simulink model "cpu2"  (R2020a)
settings: Solver=VariableStepAuto  StartTime=0.0  StopTime=10.0  RelTol=1e-3
libraries: simulink_extras x402, msbPllFoundation x1
(part 1 of 63)
settings Model: Creator=kishan  LastModifiedBy=kishan

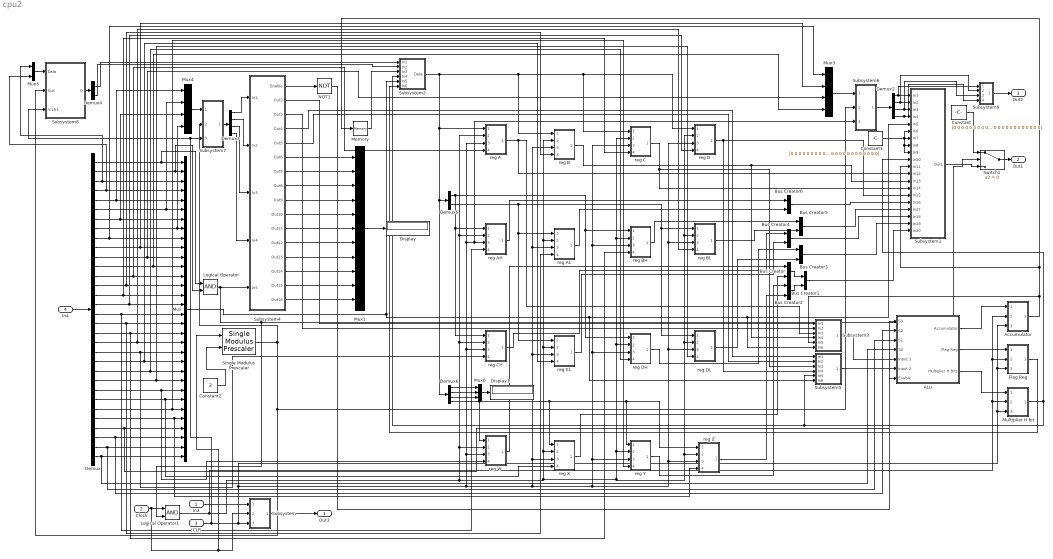
== system cpu2 ==
  In3 : Inport  OutDataTypeStr=boolean
  Clock : Inport  Port=2  OutDataTypeStr=boolean
  !CLR : Inport  Port=3  OutDataTypeStr=boolean
  In4 : Inport  Port=4
  ALU : Subsystem
  Accumulator : Subsystem
  Bus Creator{,1..6} (7 alike) : BusCreator  Inputs=2
  Constant : Constant  Value=[0 0 0 0 0 0 0 0 0 0 0 0 0 0 0 0 0 0 0 0 0 0 0 0 0 0 0 0 0 0 0 0]  OutDataTypeStr=boolean
  Constant1 : Constant  Value=[0 0 0 0 0 0 0 0 0 0 0 0 0 0 0 0 0 0 0 0 0 0 0 0 0 0 0 0 0 0 0 0]  OutDataTypeStr=boolean
  Constant2 : Constant  Value=2  OutDataTypeStr=double
  Demux : Demux  Outputs=32
  Demux2 : Demux
  Demux3 : Demux
  Demux4 : Demux  Outputs=2
  Demux5 : Demux  Outputs=2
  Demux6 : Demux
  Display : Display
  Display1 : Display
  Flag Reg : Subsystem
  Logical Operator : Logic  AllPortsSameDT=off  OutDataTypeStr=boolean
  Logical Operator1 : Logic  AllPortsSameDT=off  OutDataTypeStr=boolean
  Memory : Memory  InitialCondition=[0 0 0 0 0 0 0 0 0 0 0 0 0 0 0 0 0 0 0 0 0 0 0 0 0 0 0 0 0 0 0 0]
  Multiplier H bit : Subsystem
  Mux : Mux  Inputs=32
  Mux1 : Mux  Inputs=11
  Mux3 : Mux
  Mux4 : Mux
  Mux5 : Mux  Inputs=2
  Mux6 : Mux  Inputs=3
  NOT1 : Logic  Operator=NOT  IconShape=distinctive  AllPortsSameDT=off  OutDataTypeStr=boolean
  Single Modulus Prescaler : msbPllFoundation/Single Modulus Prescaler  ExtraBuffer=off  NBuffer=1
      settings: SourceProductBaseCode=AM
  Subsystem : Subsystem
  Subsystem1 : Subsystem
  Subsystem2 : Subsystem
  Subsystem3 : Subsystem
  Subsystem4 : Subsystem
  Subsystem5 : Subsystem
  Subsystem6 : Subsystem
  Subsystem7 : Subsystem
  Subsystem8 : Subsystem
  Subsystem9 : Subsystem
  Switch1 : Switch  Criteria=u2 > Threshold  OutDataTypeStr=boolean
  reg A : Subsystem
  reg AH : Subsystem
  reg AL : Subsystem
  reg B : Subsystem
  reg BH : Subsystem
  reg BL : Subsystem
  reg C : Subsystem
  reg CH : Subsystem
  reg CL : Subsystem
  reg D : Subsystem
  reg DH : Subsystem
  reg DL : Subsystem
  reg W : Subsystem
  reg X : Subsystem
  reg Y : Subsystem
  reg Z : Subsystem
  Out3 : Outport
  Out1 : Outport  Port=2
  Out2 : Outport  Port=3
  wires:
  Logical Operator/1 -> Logical Operator1/2, Switch1/2, Subsystem4/5(In5)
  Subsystem4/5(Out5) -> Subsystem5/2(In2)
  Demux/7 -> Mux/7, Mux4/3
  Demux/19 -> reg BH/4(Mux_in), Mux/19
  Mux/1 -> Subsystem5/6(In6), Subsystem3/6(In6), Subsystem1/5(In5), Subsystem2/5(In5)
  Subsystem5/1(Input 2) -> ALU/6(Input 2)
  Subsystem4/8(Out8) -> Mux1/3
  Subsystem4/13(Out13) -> Mux1/8
  Demux/23 -> reg DH/4(Mux_in), Mux/23
  Subsystem4/2(Out2) -> Subsystem3/1(In1)
  Accumulator/1(Out1) -> Memory/1, Subsystem1/11(In11), Subsystem3/5(In5)
  ALU/3(Multiplier H Bits) -> Multiplier H bit/1(In1)
  reg Y/1(Out1) -> Bus Creator2/1
  Demux/31 -> ALU/3(S1), Mux/31
  ALU/1(Accumulator) -> Accumulator/1(In1)
  reg Z/1(Out1) -> Bus Creator2/2
  Subsystem4/3(Out3) -> Subsystem3/2(In2)
  NOT1/1 -> ALU/7(Enable)
  Constant/1 -> Switch1/1
  Flag Reg/1(Out1) -> Subsystem2/6(In6)
  Bus Creator1/1 -> Subsystem1/20(In20)
  Demux/3 -> Mux5/1, Mux/3
  Demux/28 -> reg Z/4(Mux_in), Mux/28
  Clock/1 -> Single Modulus Prescaler/1, Subsystem/2(Clock), Logical Operator1/1
  Subsystem/1(Out1) -> Out3/1
  Subsystem4/15(Out15) -> Mux1/10
  Bus Creator/1 -> Bus Creator1/1
  reg B/1(Out1) -> Subsystem1/13(In13), Subsystem3/4(In4)
  reg AH/1(Out1) -> Bus Creator6/1
  Subsystem2/1(Data) -> reg D/1(Data), reg C/1(Data), reg B/1(Data), Demux6/1, Demux5/1, reg A/1(Data)
  Subsystem4/9(Out9) -> Mux1/4
  Demux/24 -> reg DL/4(Mux_in), Mux/24
  Demux/27 -> reg Y/4(Mux_in), Mux/27
  Subsystem4/1(Enable) -> NOT1/1
  reg C/1(Out1) -> Subsystem1/14(In14), Subsystem5/3(In3)
  Bus Creator6/1 -> Subsystem1/16(In16)
  reg BL/1(Out1) -> Bus Creator5/2
  In4/1 -> Demux/1
  Subsystem4/10(Out10) -> Mux1/5
  Subsystem4/7(Out7) -> Mux1/2
  reg DL/1(Out1) -> Bus Creator3/2
  Logical Operator1/1 -> Accumulator/2(In2), Flag Reg/2(In2), Multiplier H bit/2(In2), reg DH/2(In2), reg BH/2(In2), reg C/2(In2), reg Y/2(In2), reg Z/2(In2), reg BL/2(In2), reg D/2(In2), reg DL/2(In2), reg X/2(In2), reg CL/2(In2), reg AL/2(In2), reg B/2(In2), reg W/2(In2), reg CH/2(In2), reg AH/2(In2), reg A/2(In2)
  Bus Creator3/1 -> Subsystem1/19(In19)
  ALU/2(Flag Reg) -> Flag Reg/1(In1)
  reg W/1(Out1) -> Bus Creator/1
  Demux/15 -> reg C/4(Mux_in), Mux/15
  Demux/13 -> reg A/4(Mux_in), Mux/13
  In3/1 -> Subsystem/1(Interrupt)
  Demux/16 -> reg D/4(Mux_in), Mux/16
  Subsystem4/11(Out11) -> Mux1/6
  Bus Creator5/1 -> Subsystem1/17(In17)
  Subsystem4/14(Out14) -> Mux1/9
  Subsystem4/16(Out16) -> Mux1/11
  Demux/29 -> ALU/1(S3), Mux/29
  Subsystem4/12(Out12) -> Mux1/7
  reg D/1(Out1) -> Subsystem1/15(In15), Subsystem5/4(In4)
  Switch1/1 -> Out1/1
  Demux/11 -> Mux3/3, Mux/11
  Demux/2 -> Logical Operator/2, Mux/2
  reg CL/1(Out1) -> Bus Creator4/2
  Demux/5 -> Mux4/1, Mux/5
  Demux/20 -> reg BL/4(Mux_in), Mux/20
  Bus Creator4/1 -> Subsystem1/18(In18)
  Demux/9 -> Mux3/1, Mux/9
  Demux/1 -> Mux/1, Logical Operator/1
  Demux/14 -> reg B/4(Mux_in), Mux/14
  Demux/25 -> reg W/4(Mux_in), Mux/25
  Memory/1 -> Subsystem2/3(In3)
  Demux/26 -> reg X/4(Mux_in), Mux/26
  Demux/32 -> ALU/4(S0), Mux/32
  reg DH/1(Out1) -> Bus Creator3/1
  Demux/30 -> ALU/2(S2), Mux/30
  Multiplier H bit/1(Out1) -> Subsystem5/5(In5), Subsystem2/4(In4), Subsystem1/10(In10)
  Demux/6 -> Mux4/2, Mux/6
  Subsystem3/1(Input 1) -> ALU/5(Input 1)
  Subsystem4/6(Out6) -> Mux1/1
  Demux/10 -> Mux3/2, Mux/10
  Demux/12 -> Mux3/4, Mux/12
  Mux1/1 -> Display/1
  reg X/1(Out1) -> Bus Creator/2
  !CLR/1 -> Subsystem8/3(!CLR1), Subsystem7/3(!CLR), Accumulator/3(In3), Flag Reg/3(In3), Multiplier H bit/3(In3), reg CH/3(In3), Subsystem6/3(!CLR), reg AH/3(In3), reg A/3(In3), reg W/3(In3), reg X/3(In3), reg CL/3(In3), reg AL/3(In3), reg B/3(In3), reg DH/3(In3), reg BH/3(In3), reg C/3(In3), reg Y/3(In3), reg Z/3(In3), reg BL/3(In3), reg D/3(In3), reg DL/3(In3), Subsystem/3(Reset)
  reg A/1(Out1) -> Subsystem3/3(In3), Subsystem1/12(In12)
  Demux/8 -> Mux4/4, Mux/8
  Bus Creator2/1 -> Bus Creator1/2
  Subsystem4/4(Out4) -> Subsystem5/1(In1)
  Constant1/1 -> Subsystem1/9(In9), Subsystem1/8(In8), Subsystem1/7(In7), Subsystem1/6(In6)
  reg CH/1(Out1) -> Bus Creator4/1
  reg AL/1(Out1) -> Bus Creator6/2
  reg BH/1(Out1) -> Bus Creator5/1
  Demux/22 -> reg CL/4(Mux_in), Mux/22
  Demux/21 -> reg CH/4(Mux_in), Mux/21
  Demux/4 -> Mux5/2, Mux/4
  Demux/18 -> reg AL/4(Mux_in), Mux/18
  Subsystem1/1(Out1) -> Switch1/3
  Demux/17 -> reg AH/4(Mux_in), Mux/17
  Single Modulus Prescaler/1 -> Subsystem7/2(CLK), Subsystem8/2(CLK), Subsystem6/2(CLK)
  Constant2/1 -> Single Modulus Prescaler/2
  Mux3/1 -> Subsystem6/1(Data)
  Demux2/1 -> Subsystem1/1(In1), Subsystem9/1(In1)
  Demux2/2 -> Subsystem9/2(In2), Subsystem1/2(In2)
  Demux2/3 -> Subsystem9/3(In3), Subsystem1/3(In3)
  Demux2/4 -> Subsystem9/4(In4), Subsystem1/4(In4)
  Subsystem6/1(Out1) -> Demux2/1
  Subsystem7/1(Out1) -> Demux3/1
  Mux4/1 -> Subsystem7/1(Data)
  Demux3/1 -> Subsystem4/1(In1)
  Demux3/2 -> Subsystem4/2(In2)
  Demux3/4 -> Subsystem4/4(In4)
  Demux3/3 -> Subsystem4/3(In3)
  Mux5/1 -> Subsystem8/1(Data)
  Subsystem8/1(Q) -> Demux4/1
  Demux4/1 -> Subsystem2/1(In1)
  Demux4/2 -> Subsystem2/2(In2)
  Demux5/1 -> reg DH/1(Data), reg BH/1(Data), reg CH/1(Data), reg AH/1(Data)
  Demux5/2 -> reg DL/1(Data), reg BL/1(Data), reg CL/1(Data), reg AL/1(Data)
  Demux6/4 -> reg W/1(Data), reg X/1(Data), reg Y/1(Data), reg Z/1(Data)
  Demux6/1 -> Mux6/1
  Demux6/2 -> Mux6/2
  Demux6/3 -> Mux6/3
  Mux6/1 -> Display1/1
  Subsystem9/1(Out1) -> Out2/1

== system cpu2/ALU ==
  S3 : Inport
  S2 : Inport  Port=2
  S1 : Inport  Port=3
  S0 : Inport  Port=4
  Input 1 : Inport  Port=5
  Input 2 : Inport  Port=6
  Enable : Inport  Port=7
  Adder : Subsystem
  Comparartor : Subsystem
  Decrementer : Subsystem
  Demux : Demux  Outputs=32
  Demux1 : Demux  Outputs=32
  Incrementer : Subsystem
  Left Rotator : Subsystem
  Left shifter : Subsystem
  Logical Operator : Logic  AllPortsSameDT=off  OutDataTypeStr=boolean
  Logical Operator1 : Logic  Operator=OR  AllPortsSameDT=off  OutDataTypeStr=boolean
  Logical Operator2 : Logic  Operator=NOT  AllPortsSameDT=off  OutDataTypeStr=boolean
  Logical Operator4 : Logic  Operator=NOR  Inputs=32  AllPortsSameDT=off  OutDataTypeStr=boolean
  Logical Operator5 : Logic  Operator=NXOR  Inputs=32  AllPortsSameDT=off  OutDataTypeStr=boolean
  Multiplier : Subsystem
  Mux : Mux  Inputs=8
  Ones : Constant  Value=[1 1 1 1 1 1 1 1 1 1 1 1 1 1 1 1 1 1 1 1 1 1 1 1 1 1 1 1 1 1 1 1]  OutDataTypeStr=boolean
  Right Shifter : Subsystem
  Right rotator : Subsystem
  Subsystem7 : Subsystem
  Subtractor : Subsystem
  Zeros : Constant  Value=[0 0 0 0 0 0 0 0 0 0 0 0 0 0 0 0 0 0 0 0 0 0 0 0 0 0 0 0 0 0 0 0]  OutDataTypeStr=boolean
  Accumulator : Outport
  Flag Reg : Outport  Port=2
  Multiplier H Bits : Outport  Port=3
  wires:
  Demux/1 -> Logical Operator4/1
  Demux/4 -> Logical Operator4/4
  Logical Operator2/1 -> Subsystem7/9(In8)
  Decrementer/2(Out2) -> Subsystem7/12(In12)
  Demux1/2 -> Logical Operator5/2
  Zeros/1 -> Subsystem7/5(In9)
  Demux1/20 -> Logical Operator5/20
  Demux/26 -> Logical Operator4/26
  Left shifter/1(Out1) -> Mux/2
  Incrementer/2(Out2) -> Subsystem7/10(In10)
  Adder/2(Out2) -> Subsystem7/14(In14)
  Demux1/21 -> Logical Operator5/21
  Demux1/9 -> Logical Operator5/9
  Demux/30 -> Logical Operator4/30
  Demux1/24 -> Logical Operator5/24
  Demux/17 -> Logical Operator4/17
  Demux1/25 -> Logical Operator5/25
  Demux1/15 -> Logical Operator5/15
  Demux1/28 -> Logical Operator5/28
  Demux/23 -> Logical Operator4/23
  Left shifter/2(Out2) -> Subsystem7/11(In11)
  Logical Operator5/1 -> Mux/8
  Logical Operator1/1 -> Subsystem7/8(In6)
  Demux/16 -> Logical Operator4/16
  Demux1/5 -> Logical Operator5/5
  Demux/5 -> Logical Operator4/5
  Demux/6 -> Logical Operator4/6
  Demux1/27 -> Logical Operator5/27
  Demux1/26 -> Logical Operator5/26
  Multiplier/1(Out1) -> Multiplier H Bits/1
  Demux/29 -> Logical Operator4/29
  Demux1/23 -> Logical Operator5/23
  Demux1/10 -> Logical Operator5/10
  Ones/1 -> Subsystem7/6(In2)
  Enable/1 -> Subsystem7/21(In21)
  S3/1 -> Subsystem7/1(In1)
  Demux1/17 -> Logical Operator5/17
  Demux1/1 -> Logical Operator5/1
  Demux/22 -> Logical Operator4/22
  Demux1/30 -> Logical Operator5/30
  Demux/2 -> Logical Operator4/2
  Demux1/22 -> Logical Operator5/22
  Logical Operator/1 -> Subsystem7/7(In4)
  Subsystem7/1(Out1) -> Accumulator/1, Demux1/1, Demux/1
  Demux/25 -> Logical Operator4/25
  Demux1/6 -> Logical Operator5/6
  Subtractor/1(Out1) -> Mux/6
  Multiplier/2(Out2) -> Subsystem7/19(In19)
  Demux1/19 -> Logical Operator5/19
  Mux/1 -> Flag Reg/1
  Demux/20 -> Logical Operator4/20
  S1/1 -> Subsystem7/3(In5)
  Demux/31 -> Logical Operator4/31
  Subtractor/2(Out2) -> Subsystem7/15(In15)
  Demux/14 -> Logical Operator4/14
  S0/1 -> Subsystem7/4(In7)
  Demux/7 -> Logical Operator4/7
  Demux/11 -> Logical Operator4/11
  Demux1/13 -> Logical Operator5/13
  Demux/10 -> Logical Operator4/10
  Demux/12 -> Logical Operator4/12
  Input 1/1 -> Left Rotator/1(Input 1), Right rotator/1(Input 1), Comparartor/1(In1), Adder/1(In1), Subsystem7/16(Input 1), Left shifter/1(Input 1), Right Shifter/1(Input 1), Decrementer/1(In1), Incrementer/1(In1), Logical Operator2/1, Logical Operator/1, Logical Operator1/1, Subtractor/1(In1), Multiplier/1(In1)
  Demux/15 -> Logical Operator4/15
  S2/1 -> Subsystem7/2(In3)
  Input 2/1 -> Comparartor/2(In2), Logical Operator1/2, Logical Operator/2, Subtractor/2(In2), Adder/2(In2), Multiplier/2(In2)
  Adder/1(Out1) -> Mux/5
  Demux/18 -> Logical Operator4/18
  Demux1/12 -> Logical Operator5/12
  Demux/21 -> Logical Operator4/21
  Decrementer/1(Out1) -> Mux/3
  Demux/13 -> Logical Operator4/13
  Right Shifter/1(Out3) -> Mux/4
  Incrementer/1(Out1) -> Mux/1
  Demux1/14 -> Logical Operator5/14
  Demux1/32 -> Logical Operator5/32
  Demux/32 -> Logical Operator4/32
  Demux1/16 -> Logical Operator5/16
  Demux1/31 -> Logical Operator5/31
  Comparartor/1(Out1) -> Subsystem7/20(In20)
  Demux/3 -> Logical Operator4/3
  Logical Operator4/1 -> Mux/7
  Demux/27 -> Logical Operator4/27
  Demux1/18 -> Logical Operator5/18
  Demux/8 -> Logical Operator4/8
  Demux1/3 -> Logical Operator5/3
  Demux1/11 -> Logical Operator5/11
  Demux/9 -> Logical Operator4/9
  Demux1/7 -> Logical Operator5/7
  Demux/24 -> Logical Operator4/24
  Demux1/29 -> Logical Operator5/29
  Demux1/4 -> Logical Operator5/4
  Demux1/8 -> Logical Operator5/8
  Right Shifter/2(Out4) -> Subsystem7/13(In13)
  Demux/28 -> Logical Operator4/28
  Demux/19 -> Logical Operator4/19
  Left Rotator/1(Out4) -> Subsystem7/17(In17)
  Right rotator/1(Out2) -> Subsystem7/18(In18)

== system cpu2/Accumulator ==
  In1 : Inport
  In2 : Inport  Port=2
  In3 : Inport  Port=3
  Demux : Demux
  Mux : Mux
  Subsystem : Subsystem
  Subsystem1 : Subsystem
  Subsystem2 : Subsystem
  Subsystem3 : Subsystem
  Out1 : Outport
  wires:
  Demux/1 -> Subsystem/1(In1)
  Demux/3 -> Subsystem2/1(In1)
  Demux/2 -> Subsystem1/1(In1)
  Subsystem1/1(Out1) -> Mux/2
  Mux/1 -> Out1/1
  Subsystem/1(Out1) -> Mux/1
  In2/1 -> Subsystem/2(In2), Subsystem1/2(In2), Subsystem2/2(In2), Subsystem3/2(In2)
  In3/1 -> Subsystem/3(In3), Subsystem1/3(In3), Subsystem2/3(In3), Subsystem3/3(In3)
  Subsystem3/1(Out1) -> Mux/4
  Subsystem2/1(Out1) -> Mux/3
  In1/1 -> Demux/1
  Demux/4 -> Subsystem3/1(In1)

== system cpu2/Flag Reg ==
  In1 : Inport
  In2 : Inport  Port=2
  In3 : Inport  Port=3
  D Flip-Flop{,1..7} (8 alike) : simulink_extras/Flip Flops/D Flip-Flop
  Demux : Demux  Outputs=8
  Display : Display
  Mux : Mux  Inputs=8
  Mux1 : Mux  Inputs=8
  Out1 : Outport
  wires:
  Demux/5 -> D Flip-Flop4/1
  Mux/1 -> Out1/1
  Demux/8 -> D Flip-Flop7/1
  D Flip-Flop3/1 -> Mux/4
  Mux1/1 -> Display/1
  D Flip-Flop/1 -> Mux/1
  D Flip-Flop7/2 -> Mux1/8
  D Flip-Flop1/2 -> Mux1/2
  D Flip-Flop6/1 -> Mux/7
  In3/1 -> D Flip-Flop7/3, D Flip-Flop6/3, D Flip-Flop5/3, D Flip-Flop4/3, D Flip-Flop3/3, D Flip-Flop2/3, D Flip-Flop1/3, D Flip-Flop/3
  Demux/4 -> D Flip-Flop3/1
  D Flip-Flop4/1 -> Mux/5
  In2/1 -> D Flip-Flop7/2, D Flip-Flop6/2, D Flip-Flop5/2, D Flip-Flop4/2, D Flip-Flop3/2, D Flip-Flop2/2, D Flip-Flop/2, D Flip-Flop1/2
  D Flip-Flop4/2 -> Mux1/5
  Demux/7 -> D Flip-Flop6/1
  D Flip-Flop5/2 -> Mux1/6
  D Flip-Flop/2 -> Mux1/1
  D Flip-Flop1/1 -> Mux/2
  D Flip-Flop2/2 -> Mux1/3
  Demux/1 -> D Flip-Flop/1
  D Flip-Flop2/1 -> Mux/3
  D Flip-Flop5/1 -> Mux/6
  In1/1 -> Demux/1
  D Flip-Flop6/2 -> Mux1/7
  Demux/2 -> D Flip-Flop1/1
  Demux/6 -> D Flip-Flop5/1
  D Flip-Flop7/1 -> Mux/8
  D Flip-Flop3/2 -> Mux1/4
  Demux/3 -> D Flip-Flop2/1

== system cpu2/Multiplier H bit ==
  In1 : Inport
  In2 : Inport  Port=2
  In3 : Inport  Port=3
  Demux : Demux
  Mux : Mux
  Subsystem : Subsystem
  Subsystem1 : Subsystem
  Subsystem2 : Subsystem
  Subsystem3 : Subsystem
  Out1 : Outport
  wires:
  Demux/1 -> Subsystem/1(In1)
  Demux/3 -> Subsystem2/1(In1)
  Demux/2 -> Subsystem1/1(In1)
  Subsystem1/1(Out1) -> Mux/2
  Mux/1 -> Out1/1
  Subsystem/1(Out1) -> Mux/1
  In2/1 -> Subsystem/2(In2), Subsystem1/2(In2), Subsystem2/2(In2), Subsystem3/2(In2)
  In3/1 -> Subsystem/3(In3), Subsystem1/3(In3), Subsystem2/3(In3), Subsystem3/3(In3)
  Subsystem3/1(Out1) -> Mux/4
  Subsystem2/1(Out1) -> Mux/3
  In1/1 -> Demux/1
  Demux/4 -> Subsystem3/1(In1)

== system cpu2/Subsystem ==
  Interrupt : Inport
  Clock : Inport  Port=2
  Reset : Inport  Port=3
  Bus Creator : BusCreator  Inputs=32
  Logical Operator : Logic  AllPortsSameDT=off  OutDataTypeStr=boolean
  Logical Operator1 : Logic  Operator=NOT  AllPortsSameDT=off  OutDataTypeStr=boolean
  Subsystem1 : Subsystem
  Out1 : Outport
  wires:
  Subsystem1/19(Out19) -> Bus Creator/19
  Subsystem1/8(Out8) -> Bus Creator/8
  Subsystem1/29(Out29) -> Bus Creator/29
  Subsystem1/21(Out21) -> Bus Creator/21
  Subsystem1/5(Out5) -> Bus Creator/5
  Subsystem1/17(Out17) -> Bus Creator/17
  Subsystem1/6(Out6) -> Bus Creator/6
  Subsystem1/23(Out23) -> Bus Creator/23
  Subsystem1/24(Out24) -> Bus Creator/24
  Subsystem1/4(Out4) -> Bus Creator/4
  Subsystem1/18(Out18) -> Bus Creator/18
  Subsystem1/26(Out26) -> Bus Creator/26
  Subsystem1/12(Out12) -> Bus Creator/12
  Subsystem1/20(Out20) -> Bus Creator/20
  Subsystem1/1(Out3) -> Bus Creator/1
  Subsystem1/2(Out1) -> Bus Creator/2
  Subsystem1/14(Out14) -> Bus Creator/14
  Clock/1 -> Logical Operator/2
  Bus Creator/1 -> Out1/1
  Subsystem1/28(Out28) -> Bus Creator/28
  Subsystem1/30(Out30) -> Bus Creator/30
  Reset/1 -> Subsystem1/2(In2)
  Subsystem1/16(Out16) -> Bus Creator/16
  Subsystem1/3(Out2) -> Bus Creator/3
  Subsystem1/10(Out10) -> Bus Creator/10
  Subsystem1/25(Out25) -> Bus Creator/25
  Subsystem1/32(Out32) -> Bus Creator/32
  Subsystem1/9(Out9) -> Bus Creator/9
  Subsystem1/13(Out13) -> Bus Creator/13
  Subsystem1/22(Out22) -> Bus Creator/22
  Subsystem1/15(Out15) -> Bus Creator/15
  Subsystem1/31(Out31) -> Bus Creator/31
  Subsystem1/11(Out11) -> Bus Creator/11
  Subsystem1/27(Out27) -> Bus Creator/27
  Subsystem1/7(Out7) -> Bus Creator/7
  Logical Operator/1 -> Subsystem1/1(In1)
  Interrupt/1 -> Logical Operator1/1
  Logical Operator1/1 -> Logical Operator/1

== system cpu2/Subsystem1 ==
  In1 : Inport
  In2 : Inport  Port=2
  In3 : Inport  Port=3
  In4 : Inport  Port=4  OutDataTypeStr=boolean
  In5 : Inport  Port=5  OutDataTypeStr=boolean
  In6 : Inport  Port=6
  In7 : Inport  Port=7
  In8 : Inport  Port=8
  In9 : Inport  Port=9
  In10 : Inport  Port=10  OutDataTypeStr=boolean
  In11 : Inport  Port=11  OutDataTypeStr=boolean
  In12 : Inport  Port=12  OutDataTypeStr=boolean
  In13 : Inport  Port=13  OutDataTypeStr=boolean
  In14 : Inport  Port=14
  In15 : Inport  Port=15
  In16 : Inport  Port=16
  In17 : Inport  Port=17
  In18 : Inport  Port=18  OutDataTypeStr=boolean
  In19 : Inport  Port=19  OutDataTypeStr=boolean
  In20 : Inport  Port=20  OutDataTypeStr=boolean
  NOT : Logic  Operator=NOT  IconShape=distinctive  AllPortsSameDT=off  OutDataTypeStr=boolean
  NOT1 : Logic  Operator=NOT  IconShape=distinctive  AllPortsSameDT=off  OutDataTypeStr=boolean
  NOT2 : Logic  Operator=NOT  IconShape=distinctive  AllPortsSameDT=off  OutDataTypeStr=boolean
  Switch{1..3,5..7,9..11,16..17,19..20} (13 alike) : Switch  Criteria=u2 > Threshold  OutDataTypeStr=boolean
  Switch4 : Switch  Criteria=u2 > Threshold
  Switch8 : Switch  Criteria=u2 > Threshold
  Out1 : Outport
  wires:
  Switch19/1 -> Switch17/1
  Switch9/1 -> Switch16/3
  Switch16/1 -> Out1/1
  Switch10/1 -> Switch9/1
  Switch20/1 -> Switch17/3
  Switch17/1 -> Switch16/1
  Switch11/1 -> Switch9/3
  Switch1/1 -> Switch19/1
  Switch2/1 -> Switch19/3
  Switch3/1 -> Switch20/1
  Switch4/1 -> Switch20/3
  Switch5/1 -> Switch10/1
  Switch8/1 -> Switch11/3
  Switch6/1 -> Switch10/3
  Switch7/1 -> Switch11/1
  In1/1 -> Switch16/2
  In2/1 -> NOT/1, Switch17/2
  In3/1 -> Switch10/2, Switch19/2, NOT1/1
  NOT/1 -> Switch9/2
  NOT1/1 -> Switch11/2, Switch20/2
  In4/1 -> Switch7/2, Switch5/2, Switch3/2, NOT2/1, Switch1/2
  In5/1 -> Switch1/1
  In6/1 -> Switch1/3
  In8/1 -> Switch2/3
  In7/1 -> Switch2/1
  In10/1 -> Switch3/3
  In9/1 -> Switch3/1
  In12/1 -> Switch4/3
  In11/1 -> Switch4/1
  In14/1 -> Switch5/3
  In13/1 -> Switch5/1
  In16/1 -> Switch6/3
  In15/1 -> Switch6/1
  In18/1 -> Switch7/3
  In17/1 -> Switch7/1
  In20/1 -> Switch8/3
  In19/1 -> Switch8/1
  NOT2/1 -> Switch4/2, Switch6/2, Switch8/2, Switch2/2

== system cpu2/Subsystem2 ==
  In1 : Inport
  In2 : Inport  Port=2
  In3 : Inport  Port=3
  In4 : Inport  Port=4
  In5 : Inport  Port=5
  In6 : Inport  Port=6
  Constant1 : Constant  Value=[0 0 0 0 0 0 0 0 0 0 0 0 0 0 0 0 0 0 0 0 0 0 0 0]  OutDataTypeStr=boolean
  Mux5 : Mux  Inputs=2
  NOT : Logic  Operator=NOT  IconShape=distinctive  AllPortsSameDT=off  OutDataTypeStr=boolean
  Switch1 : Switch  Criteria=u2 > Threshold
  Switch15 : Switch  Criteria=u2 > Threshold
  Switch2 : Switch  Criteria=u2 > Threshold
  Data : Outport
  wires:
  Switch15/1 -> Data/1
  Switch1/1 -> Switch15/1
  Switch2/1 -> Switch15/3
  In1/1 -> Switch15/2
  In2/1 -> NOT/1, Switch1/2
  NOT/1 -> Switch2/2
  In3/1 -> Switch1/1
  In4/1 -> Switch1/3
  In5/1 -> Switch2/1
  Mux5/1 -> Switch2/3
  In6/1 -> Mux5/2
  Constant1/1 -> Mux5/1

== system cpu2/Subsystem3 ==
  In1 : Inport
  In2 : Inport  Port=2
  In3 : Inport  Port=3
  In4 : Inport  Port=4
  In5 : Inport  Port=5
  In6 : Inport  Port=6
  NOT : Logic  Operator=NOT  IconShape=distinctive  AllPortsSameDT=off  OutDataTypeStr=boolean
  Switch1 : Switch  Criteria=u2 > Threshold
  Switch2 : Switch  Criteria=u2 > Threshold
  Switch3 : Switch  Criteria=u2 > Threshold
  Input 1 : Outport
  wires:
  In4/1 -> Switch2/3
  In2/1 -> NOT/1, Switch2/2
  In3/1 -> Switch2/1
  Switch2/1 -> Switch3/1
  Switch1/1 -> Switch3/3
  Switch3/1 -> Input 1/1
  In1/1 -> Switch3/2
  In5/1 -> Switch1/1
  In6/1 -> Switch1/3
  NOT/1 -> Switch1/2

== system cpu2/Subsystem4 ==
  In1 : Inport
  In2 : Inport  Port=2
  In3 : Inport  Port=3
  In4 : Inport  Port=4
  In5 : Inport  Port=5
  Subsystem1 : Subsystem
  Enable : Outport
  Out2 : Outport  Port=2
  Out3 : Outport  Port=3
  Out4 : Outport  Port=4
  Out5 : Outport  Port=5
  Out6 : Outport  Port=6
  Out7 : Outport  Port=7
  Out8 : Outport  Port=8
  Out9 : Outport  Port=9
  Out10 : Outport  Port=10
  Out11 : Outport  Port=11
  Out12 : Outport  Port=12
  Out13 : Outport  Port=13
  Out14 : Outport  Port=14
  Out15 : Outport  Port=15
  Out16 : Outport  Port=16
  wires:
  Subsystem1/15(Out15) -> Out15/1
  Subsystem1/13(Out13) -> Out13/1
  Subsystem1/12(Out12) -> Out12/1
  In3/1 -> Subsystem1/3(In3)
  Subsystem1/8(Out8) -> Out8/1
  In4/1 -> Subsystem1/4(In4)
  Subsystem1/11(Out11) -> Out11/1
  In1/1 -> Subsystem1/1(In1)
  Subsystem1/10(Out10) -> Out10/1
  Subsystem1/7(Out7) -> Out7/1
  Subsystem1/6(Out6) -> Out6/1
  In2/1 -> Subsystem1/2(In2)
  Subsystem1/5(Out5) -> Out5/1
  Subsystem1/3(Out3) -> Out3/1
  Subsystem1/4(Out4) -> Out4/1
  Subsystem1/1(Out1) -> Enable/1
  Subsystem1/2(Out2) -> Out2/1
  Subsystem1/16(Out16) -> Out16/1
  Subsystem1/14(Out14) -> Out14/1
  Subsystem1/9(Out9) -> Out9/1
  In5/1 -> Subsystem1/5(In5)

== system cpu2/Subsystem5 ==
  In1 : Inport
  In2 : Inport  Port=2
  In3 : Inport  Port=3
  In4 : Inport  Port=4
  In5 : Inport  Port=5
  In6 : Inport  Port=6
  NOT : Logic  Operator=NOT  IconShape=distinctive  AllPortsSameDT=off  OutDataTypeStr=boolean
  Switch1 : Switch  Criteria=u2 > Threshold
  Switch2 : Switch  Criteria=u2 > Threshold
  Switch3 : Switch  Criteria=u2 > Threshold
  Input 2 : Outport
  wires:
  In4/1 -> Switch2/3
  In2/1 -> NOT/1, Switch2/2
  In3/1 -> Switch2/1
  Switch2/1 -> Switch3/1
  Switch1/1 -> Switch3/3
  Switch3/1 -> Input 2/1
  In1/1 -> Switch3/2
  In5/1 -> Switch1/1
  In6/1 -> Switch1/3
  NOT/1 -> Switch1/2

== system cpu2/Subsystem6 ==
  Data : Inport
  CLK : Inport  Port=2
  !CLR : Inport  Port=3
  D Flip-Flop{,1..3} (4 alike) : simulink_extras/Flip Flops/D Flip-Flop
  Demux : Demux
  Display : Display
  Mux : Mux
  Mux1 : Mux
  Out1 : Outport
  wires:
  !CLR/1 -> D Flip-Flop/3, D Flip-Flop1/3, D Flip-Flop2/3, D Flip-Flop3/3
  CLK/1 -> D Flip-Flop/2, D Flip-Flop1/2, D Flip-Flop2/2, D Flip-Flop3/2
  Demux/1 -> D Flip-Flop/1
  Demux/2 -> D Flip-Flop1/1
  Demux/3 -> D Flip-Flop2/1
  Demux/4 -> D Flip-Flop3/1
  Data/1 -> Demux/1
  D Flip-Flop/1 -> Mux/1
  D Flip-Flop1/1 -> Mux/2
  D Flip-Flop2/1 -> Mux/3
  D Flip-Flop3/1 -> Mux/4
  D Flip-Flop/2 -> Mux1/1
  D Flip-Flop1/2 -> Mux1/2
  D Flip-Flop2/2 -> Mux1/3
  D Flip-Flop3/2 -> Mux1/4
  Mux1/1 -> Display/1
  Mux/1 -> Out1/1

== system cpu2/Subsystem7 ==
  Data : Inport
  CLK : Inport  Port=2
  !CLR : Inport  Port=3
  D Flip-Flop{,1..3} (4 alike) : simulink_extras/Flip Flops/D Flip-Flop
  Demux : Demux
  Display : Display
  Mux : Mux
  Mux1 : Mux
  Out1 : Outport
  wires:
  !CLR/1 -> D Flip-Flop2/3, D Flip-Flop/3, D Flip-Flop1/3, D Flip-Flop3/3
  CLK/1 -> D Flip-Flop2/2, D Flip-Flop/2, D Flip-Flop1/2, D Flip-Flop3/2
  Demux/1 -> D Flip-Flop/1
  Demux/2 -> D Flip-Flop1/1
  Demux/3 -> D Flip-Flop2/1
  Demux/4 -> D Flip-Flop3/1
  Data/1 -> Demux/1
  D Flip-Flop/1 -> Mux/1
  D Flip-Flop1/1 -> Mux/2
  D Flip-Flop2/1 -> Mux/3
  D Flip-Flop3/1 -> Mux/4
  D Flip-Flop/2 -> Mux1/1
  D Flip-Flop1/2 -> Mux1/2
  D Flip-Flop2/2 -> Mux1/3
  D Flip-Flop3/2 -> Mux1/4
  Mux1/1 -> Display/1
  Mux/1 -> Out1/1

== system cpu2/Subsystem8 ==
  Data : Inport
  CLK : Inport  Port=2
  !CLR1 : Inport  Port=3
  D Flip-Flop2 : simulink_extras/Flip Flops/D Flip-Flop
  D Flip-Flop3 : simulink_extras/Flip Flops/D Flip-Flop
  Demux : Demux  Outputs=2
  Display : Display
  Mux : Mux  Inputs=2
  Mux1 : Mux  Inputs=2
  Q : Outport
  wires:
  Demux/1 -> D Flip-Flop2/1
  D Flip-Flop2/1 -> Mux1/1
  CLK/1 -> D Flip-Flop2/2, D Flip-Flop3/2
  !CLR1/1 -> D Flip-Flop2/3, D Flip-Flop3/3
  D Flip-Flop2/2 -> Mux/1
  D Flip-Flop3/2 -> Mux/2
  Mux/1 -> Display/1
  Mux1/1 -> Q/1
  D Flip-Flop3/1 -> Mux1/2
  Data/1 -> Demux/1
  Demux/2 -> D Flip-Flop3/1

== system cpu2/Subsystem9 ==
  In1 : Inport
  In2 : Inport  Port=2
  In3 : Inport  Port=3
  In4 : Inport  Port=4
  NOT{,1..3} (4 alike) : Logic  Operator=NOT  IconShape=distinctive  AllPortsSameDT=off  OutDataTypeStr=boolean
  NOT4 : Logic  Operator=OR  Inputs=3  IconShape=distinctive  AllPortsSameDT=off  OutDataTypeStr=boolean
  NOT5 : Logic  Inputs=3  IconShape=distinctive  AllPortsSameDT=off  OutDataTypeStr=boolean
  NOT6 : Logic  Inputs=3  IconShape=distinctive  AllPortsSameDT=off  OutDataTypeStr=boolean
  NOT7 : Logic  Inputs=4  IconShape=distinctive  AllPortsSameDT=off  OutDataTypeStr=boolean
  Out1 : Outport
  wires:
  NOT/1 -> NOT7/1, NOT6/1, NOT5/1
  NOT1/1 -> NOT5/2, NOT6/2
  In1/1 -> NOT/1
  In2/1 -> NOT7/2, NOT1/1
  In3/1 -> NOT5/3, NOT2/1
  In4/1 -> NOT6/3, NOT3/1
  NOT2/1 -> NOT7/3
  NOT3/1 -> NOT7/4
  NOT5/1 -> NOT4/1
  NOT6/1 -> NOT4/2
  NOT7/1 -> NOT4/3
  NOT4/1 -> Out1/1

== system cpu2/reg A ==
  Data : Inport
  In2 : Inport  Port=2
  In3 : Inport  Port=3
  Mux_in : Inport  Port=4
  Demux : Demux
  Memory : Memory  InitialCondition=[0 0 0 0 0 0 0 0 0 0 0 0 0 0 0 0 0 0 0 0 0 0 0 0 0 0 0 0 0 0 0 0]
  Mux : Mux
  Subsystem : Subsystem
  Subsystem1 : Subsystem
  Subsystem2 : Subsystem
  Subsystem3 : Subsystem
  Switch : Switch  Criteria=u2 > Threshold
  Out1 : Outport
  wires:
  Demux/1 -> Subsystem/1(In1)
  Demux/3 -> Subsystem2/1(In1)
  Demux/2 -> Subsystem1/1(In1)
  Subsystem1/1(Out1) -> Mux/2
  Mux/1 -> Memory/1, Out1/1
  Subsystem/1(Out1) -> Mux/1
  In2/1 -> Subsystem/2(In2), Subsystem1/2(In2), Subsystem2/2(In2), Subsystem3/2(In2)
  In3/1 -> Subsystem/3(In3), Subsystem1/3(In3), Subsystem2/3(In3), Subsystem3/3(In3)
  Subsystem3/1(Out1) -> Mux/4
  Subsystem2/1(Out1) -> Mux/3
  Demux/4 -> Subsystem3/1(In1)
  Data/1 -> Switch/3
  Switch/1 -> Demux/1
  Memory/1 -> Switch/1
  Mux_in/1 -> Switch/2

== system cpu2/reg AH ==
  note: Subsystem2
  Data : Inport
  In2 : Inport  Port=2
  In3 : Inport  Port=3
  Mux_in : Inport  Port=4
  Demux : Demux  Outputs=2
  Memory : Memory  InitialCondition=[0 0 0 0 0 0 0 0 0 0 0 0 0 0 0 0]
  Mux : Mux  Inputs=2
  Subsystem : Subsystem
  Subsystem1 : Subsystem
  Switch : Switch  Criteria=u2 > Threshold
  Out1 : Outport
  wires:
  Mux/1 -> Memory/1, Out1/1
  In3/1 -> Subsystem/3(In3), Subsystem1/3(In3)
  Demux/2 -> Subsystem1/1(In1)
  Switch/1 -> Demux/1
  Subsystem/1(Out1) -> Mux/1
  In2/1 -> Subsystem/2(In2), Subsystem1/2(In2)
  Subsystem1/1(Out1) -> Mux/2
  Demux/1 -> Subsystem/1(In1)
  Memory/1 -> Switch/1
  Data/1 -> Switch/3
  Mux_in/1 -> Switch/2

== system cpu2/reg AL ==
  note: Subsystem2
  Data : Inport
  In2 : Inport  Port=2
  In3 : Inport  Port=3
  Mux_in : Inport  Port=4
  Demux : Demux  Outputs=2
  Memory : Memory  InitialCondition=[0 0 0 0 0 0 0 0 0 0 0 0 0 0 0 0]
  Mux : Mux  Inputs=2
  Subsystem : Subsystem
  Subsystem1 : Subsystem
  Switch : Switch  Criteria=u2 > Threshold
  Out1 : Outport
  wires:
  Mux/1 -> Memory/1, Out1/1
  In3/1 -> Subsystem/3(In3), Subsystem1/3(In3)
  Demux/2 -> Subsystem1/1(In1)
  Switch/1 -> Demux/1
  Subsystem/1(Out1) -> Mux/1
  In2/1 -> Subsystem/2(In2), Subsystem1/2(In2)
  Subsystem1/1(Out1) -> Mux/2
  Demux/1 -> Subsystem/1(In1)
  Memory/1 -> Switch/1
  Data/1 -> Switch/3
  Mux_in/1 -> Switch/2

== system cpu2/reg B ==
  Data : Inport
  In2 : Inport  Port=2
  In3 : Inport  Port=3
  Mux_in : Inport  Port=4
  Demux : Demux
  Memory : Memory  InitialCondition=[0 0 0 0 0 0 0 0 0 0 0 0 0 0 0 0 0 0 0 0 0 0 0 0 0 0 0 0 0 0 0 0]
  Mux : Mux
  Subsystem : Subsystem
  Subsystem1 : Subsystem
  Subsystem2 : Subsystem
  Subsystem3 : Subsystem
  Switch : Switch  Criteria=u2 > Threshold
  Out1 : Outport
  wires:
  Demux/1 -> Subsystem/1(In1)
  Demux/3 -> Subsystem2/1(In1)
  Demux/2 -> Subsystem1/1(In1)
  Subsystem1/1(Out1) -> Mux/2
  Mux/1 -> Memory/1, Out1/1
  Subsystem/1(Out1) -> Mux/1
  In2/1 -> Subsystem/2(In2), Subsystem1/2(In2), Subsystem2/2(In2), Subsystem3/2(In2)
  In3/1 -> Subsystem/3(In3), Subsystem1/3(In3), Subsystem2/3(In3), Subsystem3/3(In3)
  Subsystem3/1(Out1) -> Mux/4
  Subsystem2/1(Out1) -> Mux/3
  Demux/4 -> Subsystem3/1(In1)
  Data/1 -> Switch/3
  Switch/1 -> Demux/1
  Memory/1 -> Switch/1
  Mux_in/1 -> Switch/2

== system cpu2/reg BH ==
  note: Subsystem2
  Data : Inport
  In2 : Inport  Port=2
  In3 : Inport  Port=3
  Mux_in : Inport  Port=4
  Demux : Demux  Outputs=2
  Memory : Memory  InitialCondition=[0 0 0 0 0 0 0 0 0 0 0 0 0 0 0 0]
  Mux : Mux  Inputs=2
  Subsystem : Subsystem
  Subsystem1 : Subsystem
  Switch : Switch  Criteria=u2 > Threshold
  Out1 : Outport
  wires:
  Mux/1 -> Memory/1, Out1/1
  In3/1 -> Subsystem/3(In3), Subsystem1/3(In3)
  Demux/2 -> Subsystem1/1(In1)
  Switch/1 -> Demux/1
  Subsystem/1(Out1) -> Mux/1
  In2/1 -> Subsystem/2(In2), Subsystem1/2(In2)
  Subsystem1/1(Out1) -> Mux/2
  Demux/1 -> Subsystem/1(In1)
  Memory/1 -> Switch/1
  Data/1 -> Switch/3
  Mux_in/1 -> Switch/2

== system cpu2/reg BL ==
  note: Subsystem2
  Data : Inport
  In2 : Inport  Port=2
  In3 : Inport  Port=3
  Mux_in : Inport  Port=4
  Demux : Demux  Outputs=2
  Memory : Memory  InitialCondition=[0 0 0 0 0 0 0 0 0 0 0 0 0 0 0 0]
  Mux : Mux  Inputs=2
  Subsystem : Subsystem
  Subsystem1 : Subsystem
  Switch : Switch  Criteria=u2 > Threshold
  Out1 : Outport
  wires:
  Mux/1 -> Memory/1, Out1/1
  In3/1 -> Subsystem/3(In3), Subsystem1/3(In3)
  Demux/2 -> Subsystem1/1(In1)
  Switch/1 -> Demux/1
  Subsystem/1(Out1) -> Mux/1
  In2/1 -> Subsystem/2(In2), Subsystem1/2(In2)
  Subsystem1/1(Out1) -> Mux/2
  Demux/1 -> Subsystem/1(In1)
  Memory/1 -> Switch/1
  Data/1 -> Switch/3
  Mux_in/1 -> Switch/2

== system cpu2/reg C ==
  Data : Inport
  In2 : Inport  Port=2
  In3 : Inport  Port=3
  Mux_in : Inport  Port=4
  Demux : Demux
  Memory : Memory  InitialCondition=[0 0 0 0 0 0 0 0 0 0 0 0 0 0 0 0 0 0 0 0 0 0 0 0 0 0 0 0 0 0 0 0]
  Mux : Mux
  Subsystem : Subsystem
  Subsystem1 : Subsystem
  Subsystem2 : Subsystem
  Subsystem3 : Subsystem
  Switch : Switch  Criteria=u2 > Threshold
  Out1 : Outport
  wires:
  Demux/1 -> Subsystem/1(In1)
  Demux/3 -> Subsystem2/1(In1)
  Demux/2 -> Subsystem1/1(In1)
  Subsystem1/1(Out1) -> Mux/2
  Mux/1 -> Memory/1, Out1/1
  Subsystem/1(Out1) -> Mux/1
  In2/1 -> Subsystem/2(In2), Subsystem1/2(In2), Subsystem2/2(In2), Subsystem3/2(In2)
  In3/1 -> Subsystem/3(In3), Subsystem1/3(In3), Subsystem2/3(In3), Subsystem3/3(In3)
  Subsystem3/1(Out1) -> Mux/4
  Subsystem2/1(Out1) -> Mux/3
  Demux/4 -> Subsystem3/1(In1)
  Data/1 -> Switch/3
  Switch/1 -> Demux/1
  Memory/1 -> Switch/1
  Mux_in/1 -> Switch/2

== system cpu2/reg CH ==
  note: Subsystem2
  Data : Inport
  In2 : Inport  Port=2
  In3 : Inport  Port=3
  Mux_in : Inport  Port=4
  Demux : Demux  Outputs=2
  Memory : Memory  InitialCondition=[0 0 0 0 0 0 0 0 0 0 0 0 0 0 0 0]
  Mux : Mux  Inputs=2
  Subsystem : Subsystem
  Subsystem1 : Subsystem
  Switch : Switch  Criteria=u2 > Threshold
  Out1 : Outport
  wires:
  Mux/1 -> Memory/1, Out1/1
  In3/1 -> Subsystem/3(In3), Subsystem1/3(In3)
  Demux/2 -> Subsystem1/1(In1)
  Switch/1 -> Demux/1
  Subsystem/1(Out1) -> Mux/1
  In2/1 -> Subsystem/2(In2), Subsystem1/2(In2)
  Subsystem1/1(Out1) -> Mux/2
  Demux/1 -> Subsystem/1(In1)
  Memory/1 -> Switch/1
  Data/1 -> Switch/3
  Mux_in/1 -> Switch/2

== system cpu2/reg CL ==
  note: Subsystem2
  Data : Inport
  In2 : Inport  Port=2
  In3 : Inport  Port=3
  Mux_in : Inport  Port=4
  Demux : Demux  Outputs=2
  Memory : Memory  InitialCondition=[0 0 0 0 0 0 0 0 0 0 0 0 0 0 0 0]
  Mux : Mux  Inputs=2
  Subsystem : Subsystem
  Subsystem1 : Subsystem
  Switch : Switch  Criteria=u2 > Threshold
  Out1 : Outport
  wires:
  Mux/1 -> Memory/1, Out1/1
  In3/1 -> Subsystem/3(In3), Subsystem1/3(In3)
  Demux/2 -> Subsystem1/1(In1)
  Switch/1 -> Demux/1
  Subsystem/1(Out1) -> Mux/1
  In2/1 -> Subsystem/2(In2), Subsystem1/2(In2)
  Subsystem1/1(Out1) -> Mux/2
  Demux/1 -> Subsystem/1(In1)
  Memory/1 -> Switch/1
  Data/1 -> Switch/3
  Mux_in/1 -> Switch/2

== system cpu2/reg D ==
  Data : Inport
  In2 : Inport  Port=2
  In3 : Inport  Port=3
  Mux_in : Inport  Port=4
  Demux : Demux
  Memory : Memory  InitialCondition=[0 0 0 0 0 0 0 0 0 0 0 0 0 0 0 0 0 0 0 0 0 0 0 0 0 0 0 0 0 0 0 0]
  Mux : Mux
  Subsystem : Subsystem
  Subsystem1 : Subsystem
  Subsystem2 : Subsystem
  Subsystem3 : Subsystem
  Switch : Switch  Criteria=u2 > Threshold
  Out1 : Outport
  wires:
  Demux/1 -> Subsystem/1(In1)
  Demux/3 -> Subsystem2/1(In1)
  Demux/2 -> Subsystem1/1(In1)
  Subsystem1/1(Out1) -> Mux/2
  Mux/1 -> Memory/1, Out1/1
  Subsystem/1(Out1) -> Mux/1
  In2/1 -> Subsystem/2(In2), Subsystem1/2(In2), Subsystem2/2(In2), Subsystem3/2(In2)
  In3/1 -> Subsystem/3(In3), Subsystem1/3(In3), Subsystem2/3(In3), Subsystem3/3(In3)
  Subsystem3/1(Out1) -> Mux/4
  Subsystem2/1(Out1) -> Mux/3
  Demux/4 -> Subsystem3/1(In1)
  Data/1 -> Switch/3
  Switch/1 -> Demux/1
  Memory/1 -> Switch/1
  Mux_in/1 -> Switch/2

== system cpu2/reg DH ==
  note: Subsystem2
  Data : Inport
  In2 : Inport  Port=2
  In3 : Inport  Port=3
  Mux_in : Inport  Port=4
  Demux : Demux  Outputs=2
  Memory : Memory  InitialCondition=[0 0 0 0 0 0 0 0 0 0 0 0 0 0 0 0]
  Mux : Mux  Inputs=2
  Subsystem : Subsystem
  Subsystem1 : Subsystem
  Switch : Switch  Criteria=u2 > Threshold
  Out1 : Outport
  wires:
  Mux/1 -> Memory/1, Out1/1
  In3/1 -> Subsystem/3(In3), Subsystem1/3(In3)
  Demux/2 -> Subsystem1/1(In1)
  Switch/1 -> Demux/1
  Subsystem/1(Out1) -> Mux/1
  In2/1 -> Subsystem/2(In2), Subsystem1/2(In2)
  Subsystem1/1(Out1) -> Mux/2
  Demux/1 -> Subsystem/1(In1)
  Memory/1 -> Switch/1
  Data/1 -> Switch/3
  Mux_in/1 -> Switch/2

== system cpu2/reg DL ==
  note: Subsystem2
  Data : Inport
  In2 : Inport  Port=2
  In3 : Inport  Port=3
  Mux_in : Inport  Port=4
  Demux : Demux  Outputs=2
  Memory : Memory  InitialCondition=[0 0 0 0 0 0 0 0 0 0 0 0 0 0 0 0]
  Mux : Mux  Inputs=2
  Subsystem : Subsystem
  Subsystem1 : Subsystem
  Switch : Switch  Criteria=u2 > Threshold
  Out1 : Outport
  wires:
  Mux/1 -> Memory/1, Out1/1
  In3/1 -> Subsystem/3(In3), Subsystem1/3(In3)
  Demux/2 -> Subsystem1/1(In1)
  Switch/1 -> Demux/1
  Subsystem/1(Out1) -> Mux/1
  In2/1 -> Subsystem/2(In2), Subsystem1/2(In2)
  Subsystem1/1(Out1) -> Mux/2
  Demux/1 -> Subsystem/1(In1)
  Memory/1 -> Switch/1
  Data/1 -> Switch/3
  Mux_in/1 -> Switch/2

== system cpu2/reg W ==
  Data : Inport
  In2 : Inport  Port=2
  In3 : Inport  Port=3
  Mux_in : Inport  Port=4
  D Flip-Flop{,1..7} (8 alike) : simulink_extras/Flip Flops/D Flip-Flop
  Demux : Demux  Outputs=8
  Display : Display
  Memory : Memory  InitialCondition=[0 0 0 0 0 0 0 0]
  Mux : Mux  Inputs=8
  Mux1 : Mux  Inputs=8
  Switch : Switch  Criteria=u2 > Threshold
  Out1 : Outport
  wires:
  Demux/5 -> D Flip-Flop4/1
  Demux/8 -> D Flip-Flop7/1
  D Flip-Flop3/1 -> Mux/4
  Mux1/1 -> Display/1
  D Flip-Flop/1 -> Mux/1
  D Flip-Flop7/2 -> Mux1/8
  D Flip-Flop1/2 -> Mux1/2
  D Flip-Flop6/1 -> Mux/7
  In3/1 -> D Flip-Flop7/3, D Flip-Flop6/3, D Flip-Flop5/3, D Flip-Flop4/3, D Flip-Flop3/3, D Flip-Flop2/3, D Flip-Flop1/3, D Flip-Flop/3
  Demux/4 -> D Flip-Flop3/1
  D Flip-Flop4/1 -> Mux/5
  In2/1 -> D Flip-Flop7/2, D Flip-Flop6/2, D Flip-Flop5/2, D Flip-Flop4/2, D Flip-Flop3/2, D Flip-Flop2/2, D Flip-Flop/2, D Flip-Flop1/2
  D Flip-Flop4/2 -> Mux1/5
  Demux/7 -> D Flip-Flop6/1
  D Flip-Flop5/2 -> Mux1/6
  D Flip-Flop/2 -> Mux1/1
  D Flip-Flop1/1 -> Mux/2
  D Flip-Flop2/2 -> Mux1/3
  Demux/1 -> D Flip-Flop/1
  D Flip-Flop2/1 -> Mux/3
  D Flip-Flop5/1 -> Mux/6
  Switch/1 -> Demux/1
  D Flip-Flop6/2 -> Mux1/7
  Demux/2 -> D Flip-Flop1/1
  Demux/6 -> D Flip-Flop5/1
  D Flip-Flop7/1 -> Mux/8
  D Flip-Flop3/2 -> Mux1/4
  Demux/3 -> D Flip-Flop2/1
  Memory/1 -> Switch/1
  Mux/1 -> Memory/1, Out1/1
  Data/1 -> Switch/3
  Mux_in/1 -> Switch/2

== system cpu2/reg X ==
  Data : Inport
  In2 : Inport  Port=2
  In3 : Inport  Port=3
  Mux_in : Inport  Port=4
  D Flip-Flop{,1..7} (8 alike) : simulink_extras/Flip Flops/D Flip-Flop
  Demux : Demux  Outputs=8
  Display : Display
  Memory : Memory  InitialCondition=[0 0 0 0 0 0 0 0]
  Mux : Mux  Inputs=8
  Mux1 : Mux  Inputs=8
  Switch : Switch  Criteria=u2 > Threshold
  Out1 : Outport
  wires:
  Demux/5 -> D Flip-Flop4/1
  Demux/8 -> D Flip-Flop7/1
  D Flip-Flop3/1 -> Mux/4
  Mux1/1 -> Display/1
  D Flip-Flop/1 -> Mux/1
  D Flip-Flop7/2 -> Mux1/8
  D Flip-Flop1/2 -> Mux1/2
  D Flip-Flop6/1 -> Mux/7
  In3/1 -> D Flip-Flop7/3, D Flip-Flop6/3, D Flip-Flop5/3, D Flip-Flop4/3, D Flip-Flop3/3, D Flip-Flop2/3, D Flip-Flop1/3, D Flip-Flop/3
  Demux/4 -> D Flip-Flop3/1
  D Flip-Flop4/1 -> Mux/5
  In2/1 -> D Flip-Flop7/2, D Flip-Flop6/2, D Flip-Flop5/2, D Flip-Flop4/2, D Flip-Flop3/2, D Flip-Flop2/2, D Flip-Flop/2, D Flip-Flop1/2
  D Flip-Flop4/2 -> Mux1/5
  Demux/7 -> D Flip-Flop6/1
  D Flip-Flop5/2 -> Mux1/6
  D Flip-Flop/2 -> Mux1/1
  D Flip-Flop1/1 -> Mux/2
  D Flip-Flop2/2 -> Mux1/3
  Demux/1 -> D Flip-Flop/1
  D Flip-Flop2/1 -> Mux/3
  D Flip-Flop5/1 -> Mux/6
  Switch/1 -> Demux/1
  D Flip-Flop6/2 -> Mux1/7
  Demux/2 -> D Flip-Flop1/1
  Demux/6 -> D Flip-Flop5/1
  D Flip-Flop7/1 -> Mux/8
  D Flip-Flop3/2 -> Mux1/4
  Demux/3 -> D Flip-Flop2/1
  Memory/1 -> Switch/1
  Mux/1 -> Memory/1, Out1/1
  Data/1 -> Switch/3
  Mux_in/1 -> Switch/2

== system cpu2/reg Y ==
  Data : Inport
  In2 : Inport  Port=2
  In3 : Inport  Port=3
  Mux_in : Inport  Port=4
  D Flip-Flop{,1..7} (8 alike) : simulink_extras/Flip Flops/D Flip-Flop
  Demux : Demux  Outputs=8
  Display : Display
  Memory : Memory  InitialCondition=[0 0 0 0 0 0 0 0]
  Mux : Mux  Inputs=8
  Mux1 : Mux  Inputs=8
  Switch : Switch  Criteria=u2 > Threshold
  Out1 : Outport
  wires:
  Demux/5 -> D Flip-Flop4/1
  Demux/8 -> D Flip-Flop7/1
  D Flip-Flop3/1 -> Mux/4
  Mux1/1 -> Display/1
  D Flip-Flop/1 -> Mux/1
  D Flip-Flop7/2 -> Mux1/8
  D Flip-Flop1/2 -> Mux1/2
  D Flip-Flop6/1 -> Mux/7
  In3/1 -> D Flip-Flop7/3, D Flip-Flop6/3, D Flip-Flop5/3, D Flip-Flop4/3, D Flip-Flop3/3, D Flip-Flop2/3, D Flip-Flop1/3, D Flip-Flop/3
  Demux/4 -> D Flip-Flop3/1
  D Flip-Flop4/1 -> Mux/5
  In2/1 -> D Flip-Flop7/2, D Flip-Flop6/2, D Flip-Flop5/2, D Flip-Flop4/2, D Flip-Flop3/2, D Flip-Flop2/2, D Flip-Flop/2, D Flip-Flop1/2
  D Flip-Flop4/2 -> Mux1/5
  Demux/7 -> D Flip-Flop6/1
  D Flip-Flop5/2 -> Mux1/6
  D Flip-Flop/2 -> Mux1/1
  D Flip-Flop1/1 -> Mux/2
  D Flip-Flop2/2 -> Mux1/3
  Demux/1 -> D Flip-Flop/1
  D Flip-Flop2/1 -> Mux/3
  D Flip-Flop5/1 -> Mux/6
  Switch/1 -> Demux/1
  D Flip-Flop6/2 -> Mux1/7
  Demux/2 -> D Flip-Flop1/1
  Demux/6 -> D Flip-Flop5/1
  D Flip-Flop7/1 -> Mux/8
  D Flip-Flop3/2 -> Mux1/4
  Demux/3 -> D Flip-Flop2/1
  Memory/1 -> Switch/1
  Mux/1 -> Memory/1, Out1/1
  Data/1 -> Switch/3
  Mux_in/1 -> Switch/2

== system cpu2/reg Z ==
  Data : Inport
  In2 : Inport  Port=2
  In3 : Inport  Port=3
  Mux_in : Inport  Port=4
  D Flip-Flop{,1..7} (8 alike) : simulink_extras/Flip Flops/D Flip-Flop
  Demux : Demux  Outputs=8
  Display : Display
  Memory : Memory  InitialCondition=[0 0 0 0 0 0 0 0]
  Mux : Mux  Inputs=8
  Mux1 : Mux  Inputs=8
  Switch : Switch  Criteria=u2 > Threshold
  Out1 : Outport
  wires:
  Demux/5 -> D Flip-Flop4/1
  Demux/8 -> D Flip-Flop7/1
  D Flip-Flop3/1 -> Mux/4
  Mux1/1 -> Display/1
  D Flip-Flop/1 -> Mux/1
  D Flip-Flop7/2 -> Mux1/8
  D Flip-Flop1/2 -> Mux1/2
  D Flip-Flop6/1 -> Mux/7
  In3/1 -> D Flip-Flop7/3, D Flip-Flop6/3, D Flip-Flop5/3, D Flip-Flop4/3, D Flip-Flop3/3, D Flip-Flop2/3, D Flip-Flop1/3, D Flip-Flop/3
  Demux/4 -> D Flip-Flop3/1
  D Flip-Flop4/1 -> Mux/5
  In2/1 -> D Flip-Flop7/2, D Flip-Flop6/2, D Flip-Flop5/2, D Flip-Flop4/2, D Flip-Flop3/2, D Flip-Flop2/2, D Flip-Flop/2, D Flip-Flop1/2
  D Flip-Flop4/2 -> Mux1/5
  Demux/7 -> D Flip-Flop6/1
  D Flip-Flop5/2 -> Mux1/6
  D Flip-Flop/2 -> Mux1/1
  D Flip-Flop1/1 -> Mux/2
  D Flip-Flop2/2 -> Mux1/3
  Demux/1 -> D Flip-Flop/1
  D Flip-Flop2/1 -> Mux/3
  D Flip-Flop5/1 -> Mux/6
  Switch/1 -> Demux/1
  D Flip-Flop6/2 -> Mux1/7
  Demux/2 -> D Flip-Flop1/1
  Demux/6 -> D Flip-Flop5/1
  D Flip-Flop7/1 -> Mux/8
  D Flip-Flop3/2 -> Mux1/4
  Demux/3 -> D Flip-Flop2/1
  Memory/1 -> Switch/1
  Mux/1 -> Memory/1, Out1/1
  Data/1 -> Switch/3
  Mux_in/1 -> Switch/2

== system cpu2/ALU/Adder ==
  In1 : Inport
  In2 : Inport  Port=2
  Subsystem : Subsystem
  Zeros1 : Constant  Value=0  OutDataTypeStr=boolean
  Out1 : Outport
  Out2 : Outport  Port=2
  wires:
  Subsystem/2(Out2) -> Out2/1
  In2/1 -> Subsystem/3(In3)
  Zeros1/1 -> Subsystem/2(In2)
  In1/1 -> Subsystem/1(In1)
  Subsystem/1(Out1) -> Out1/1

== system cpu2/ALU/Comparartor ==
  In1 : Inport
  In2 : Inport  Port=2
  Comparator : Subsystem
  Comparator1 : Subsystem
  Comparator2 : Subsystem
  Comparator3 : Subsystem
  Demux : Demux
  Demux1 : Demux
  Display : Display
  Logical Operator : Logic  Operator=OR  Inputs=4  AllPortsSameDT=off  OutDataTypeStr=boolean
  Logical Operator1 : Logic  Inputs=4  AllPortsSameDT=off  OutDataTypeStr=boolean
  Logical Operator2 : Logic  AllPortsSameDT=off  OutDataTypeStr=boolean
  Logical Operator3 : Logic  Inputs=3  AllPortsSameDT=off  OutDataTypeStr=boolean
  Logical Operator4 : Logic  Inputs=4  AllPortsSameDT=off  OutDataTypeStr=boolean
  Logical Operator5 : Logic  Operator=NOR  AllPortsSameDT=off  OutDataTypeStr=boolean
  Mux : Mux
  Mux1 : Mux
  Zeros1 : Constant  Value=[0 0 0 0 0 0 0 0 0 0 0 0 0 0 0 0 0 0 0 0 0 0 0 0 0 0 0 0 0]  OutDataTypeStr=boolean
  Out1 : Outport
  wires:
  Zeros1/1 -> Mux/4
  Mux/1 -> Out1/1
  In1/1 -> Demux/1
  In2/1 -> Demux1/1
  Demux/1 -> Comparator/1(In1)
  Demux/2 -> Comparator1/1(In1)
  Demux/3 -> Comparator2/1(In1)
  Demux/4 -> Comparator3/1(In1)
  Demux1/1 -> Comparator/2(In2)
  Demux1/2 -> Comparator1/2(In2)
  Demux1/3 -> Comparator2/2(In2)
  Demux1/4 -> Comparator3/2(In2)
  Comparator/2(Out2) -> Logical Operator1/1, Logical Operator4/1, Logical Operator3/1, Logical Operator2/1
  Comparator1/2(Out2) -> Logical Operator4/2, Logical Operator3/2, Logical Operator1/2
  Comparator2/2(Out2) -> Logical Operator4/3, Logical Operator1/3
  Comparator3/2(Out2) -> Logical Operator1/4
  Logical Operator1/1 -> Logical Operator5/2, Mux/2
  Mux1/1 -> Display/1
  Comparator/1(Out1) -> Logical Operator/1
  Comparator1/1(Out1) -> Logical Operator2/2
  Logical Operator2/1 -> Logical Operator/2
  Comparator2/1(Out1) -> Logical Operator3/3
  Logical Operator3/1 -> Logical Operator/3
  Comparator3/1(Out1) -> Logical Operator4/4
  Logical Operator4/1 -> Logical Operator/4
  Logical Operator/1 -> Logical Operator5/1, Mux/1
  Comparator/3(Out3) -> Mux1/1
  Comparator1/3(Out3) -> Mux1/2
  Comparator2/3(Out3) -> Mux1/3
  Comparator3/3(Out3) -> Mux1/4
  Logical Operator5/1 -> Mux/3

== system cpu2/ALU/Decrementer ==
  In1 : Inport
  Subtractor1 : Subsystem
  Zeros1 : Constant  Value=[0 0 0 0 0 0 0 0 0 0 0 0 0 0 0 0 0 0 0 0 0 0 0 0 0 0 0 0 0 0 0 1]
  Out1 : Outport
  Out2 : Outport  Port=2
  wires:
  Zeros1/1 -> Subtractor1/2(In2)
  In1/1 -> Subtractor1/1(In1)
  Subtractor1/1(Out1) -> Out1/1
  Subtractor1/2(Out2) -> Out2/1

== system cpu2/ALU/Incrementer ==
  In1 : Inport
  Incrementer : Subsystem
  Zeros1 : Constant  Value=[0 0 0 0 0 0 0 0 0 0 0 0 0 0 0 0 0 0 0 0 0 0 0 0 0 0 0 0 0 0 0 1]  OutDataTypeStr=boolean
  Out1 : Outport
  Out2 : Outport  Port=2
  wires:
  Zeros1/1 -> Incrementer/2(In2)
  In1/1 -> Incrementer/1(In1)
  Incrementer/2(Out2) -> Out2/1
  Incrementer/1(Out1) -> Out1/1

== system cpu2/ALU/Left Rotator ==
  Input 1 : Inport
  Demux : Demux  Outputs=32
  Mux : Mux  Inputs=32
  Out4 : Outport
  wires:
  Input 1/1 -> Demux/1
  Mux/1 -> Out4/1
  Demux/1 -> Mux/2
  Demux/2 -> Mux/3
  Demux/3 -> Mux/4
  Demux/4 -> Mux/5
  Demux/5 -> Mux/6
  Demux/6 -> Mux/7
  Demux/7 -> Mux/8
  Demux/8 -> Mux/9
  Demux/9 -> Mux/10
  Demux/10 -> Mux/11
  Demux/11 -> Mux/12
  Demux/12 -> Mux/13
  Demux/13 -> Mux/14
  Demux/14 -> Mux/15
  Demux/15 -> Mux/16
  Demux/16 -> Mux/17
  Demux/17 -> Mux/18
  Demux/18 -> Mux/19
  Demux/19 -> Mux/20
  Demux/20 -> Mux/21
  Demux/21 -> Mux/22
  Demux/22 -> Mux/23
  Demux/23 -> Mux/24
  Demux/24 -> Mux/25
  Demux/25 -> Mux/26
  Demux/26 -> Mux/27
  Demux/27 -> Mux/28
  Demux/28 -> Mux/29
  Demux/29 -> Mux/30
  Demux/30 -> Mux/31
  Demux/31 -> Mux/32
  Demux/32 -> Mux/1

== system cpu2/ALU/Left shifter ==
  Input 1 : Inport
  Demux : Demux  Outputs=32
  Mux : Mux  Inputs=32
  Zeros1 : Constant  Value=0  OutDataTypeStr=boolean
  Out1 : Outport
  Out2 : Outport  Port=2
  wires:
  Zeros1/1 -> Mux/32
  Input 1/1 -> Demux/1
  Mux/1 -> Out2/1
  Demux/1 -> Out1/1
  Demux/2 -> Mux/1
  Demux/3 -> Mux/2
  Demux/4 -> Mux/3
  Demux/5 -> Mux/4
  Demux/6 -> Mux/5
  Demux/7 -> Mux/6
  Demux/8 -> Mux/7
  Demux/9 -> Mux/8
  Demux/10 -> Mux/9
  Demux/11 -> Mux/10
  Demux/12 -> Mux/11
  Demux/13 -> Mux/12
  Demux/14 -> Mux/13
  Demux/15 -> Mux/14
  Demux/16 -> Mux/15
  Demux/17 -> Mux/16
  Demux/18 -> Mux/17
  Demux/19 -> Mux/18
  Demux/20 -> Mux/19
  Demux/21 -> Mux/20
  Demux/22 -> Mux/21
  Demux/23 -> Mux/22
  Demux/24 -> Mux/23
  Demux/25 -> Mux/24
  Demux/26 -> Mux/25
  Demux/27 -> Mux/26
  Demux/28 -> Mux/27
  Demux/29 -> Mux/28
  Demux/30 -> Mux/29
  Demux/31 -> Mux/30
  Demux/32 -> Mux/31

== system cpu2/ALU/Multiplier ==
  In1 : Inport
  In2 : Inport  Port=2
  Constant : Constant  Value=0  OutDataTypeStr=boolean
  Constant1 : Constant  Value=0  OutDataTypeStr=boolean
  Constant2 : Constant  Value=[0 0 0 0 0 0 0 0 0 0 0 0 0 0 0]  OutDataTypeStr=boolean
  Demux : Demux  Outputs=2
  Demux1 : Demux  Outputs=2
  Demux2 : Demux  Outputs=2
  Display : Display
  Logical Operator : Logic  AllPortsSameDT=off  OutDataTypeStr=boolean
  Logical Operator1 : Logic  Operator=XOR  AllPortsSameDT=off  OutDataTypeStr=boolean
  Mux{,1..3} (4 alike) : Mux  Inputs=2
  Mux4 : Mux  Inputs=3
  Subsystem : Subsystem
  Subsystem1 : Subsystem
  Subsystem2 : Subsystem
  Subsystem3 : Subsystem
  Subsystem4 : Subsystem
  Subsystem5 : Subsystem
  Subsystem7 : Subsystem
  Out1 : Outport
  Out2 : Outport  Port=2
  wires:
  Constant1/1 -> Subsystem4/2(In2)
  Subsystem3/1(Out1) -> Mux2/2
  Logical Operator/1 -> Subsystem5/2(In2)
  Subsystem3/2(Out2) -> Mux4/3
  Subsystem5/2(Out2) -> Mux4/1
  Demux/2 -> Subsystem3/1(In1), Subsystem2/1(In1)
  Mux1/1 -> Subsystem/3(In3)
  Mux3/1 -> Subsystem5/3(In3)
  Subsystem4/1(Out1) -> Logical Operator/2, Logical Operator1/2
  Logical Operator1/1 -> Mux3/2
  Subsystem2/1(Out1) -> Mux1/1
  Subsystem/1(Out1) -> Logical Operator/1, Logical Operator1/1
  Subsystem5/1(Out1) -> Display/1
  In1/1 -> Demux/1
  Demux1/2 -> Subsystem1/2(In2), Subsystem3/2(In2)
  Constant/1 -> Subsystem/2(In2)
  Subsystem7/1(Out1) -> Subsystem5/1(In1)
  In2/1 -> Demux1/1
  Subsystem7/2(Out2) -> Mux2/1
  Subsystem4/2(Out2) -> Mux4/2
  Subsystem/2(Out2) -> Subsystem4/1(In1)
  Demux/1 -> Subsystem1/1(In1), Subsystem7/1(In1)
  Subsystem1/2(Out2) -> Mux/2
  Demux1/1 -> Subsystem7/2(In2), Subsystem2/2(In2)
  Constant2/1 -> Mux3/1
  Subsystem2/2(Out2) -> Mux1/2
  Mux/1 -> Subsystem/1(In1)
  Mux2/1 -> Subsystem4/3(In3)
  Subsystem1/1(Out1) -> Mux/1
  Mux4/1 -> Demux2/1
  Demux2/1 -> Out1/1
  Demux2/2 -> Out2/1

== system cpu2/ALU/Right Shifter ==
  Input 1 : Inport
  Demux : Demux  Outputs=32
  Mux : Mux  Inputs=32
  Zeros2 : Constant  Value=0  OutDataTypeStr=boolean
  Out3 : Outport
  Out4 : Outport  Port=2
  wires:
  Input 1/1 -> Demux/1
  Mux/1 -> Out4/1
  Demux/1 -> Mux/2
  Demux/2 -> Mux/3
  Demux/3 -> Mux/4
  Demux/4 -> Mux/5
  Demux/5 -> Mux/6
  Demux/6 -> Mux/7
  Demux/7 -> Mux/8
  Demux/8 -> Mux/9
  Demux/9 -> Mux/10
  Demux/10 -> Mux/11
  Demux/11 -> Mux/12
  Demux/12 -> Mux/13
  Demux/13 -> Mux/14
  Demux/14 -> Mux/15
  Demux/15 -> Mux/16
  Demux/16 -> Mux/17
  Demux/17 -> Mux/18
  Demux/18 -> Mux/19
  Demux/19 -> Mux/20
  Demux/20 -> Mux/21
  Demux/21 -> Mux/22
  Demux/22 -> Mux/23
  Demux/23 -> Mux/24
  Demux/24 -> Mux/25
  Demux/25 -> Mux/26
  Demux/26 -> Mux/27
  Demux/27 -> Mux/28
  Demux/28 -> Mux/29
  Demux/29 -> Mux/30
  Demux/30 -> Mux/31
  Demux/31 -> Mux/32
  Zeros2/1 -> Mux/1
  Demux/32 -> Out3/1

== system cpu2/ALU/Right rotator ==
  Input 1 : Inport
  Demux : Demux  Outputs=32
  Mux : Mux  Inputs=32
  Out2 : Outport
  wires:
  Input 1/1 -> Demux/1
  Mux/1 -> Out2/1
  Demux/2 -> Mux/1
  Demux/3 -> Mux/2
  Demux/4 -> Mux/3
  Demux/5 -> Mux/4
  Demux/6 -> Mux/5
  Demux/7 -> Mux/6
  Demux/8 -> Mux/7
  Demux/9 -> Mux/8
  Demux/10 -> Mux/9
  Demux/11 -> Mux/10
  Demux/12 -> Mux/11
  Demux/13 -> Mux/12
  Demux/14 -> Mux/13
  Demux/15 -> Mux/14
  Demux/16 -> Mux/15
  Demux/17 -> Mux/16
  Demux/18 -> Mux/17
  Demux/19 -> Mux/18
  Demux/20 -> Mux/19
  Demux/21 -> Mux/20
  Demux/22 -> Mux/21
  Demux/23 -> Mux/22
  Demux/24 -> Mux/23
  Demux/25 -> Mux/24
  Demux/26 -> Mux/25
  Demux/27 -> Mux/26
  Demux/28 -> Mux/27
  Demux/29 -> Mux/28
  Demux/30 -> Mux/29
  Demux/31 -> Mux/30
  Demux/32 -> Mux/31
  Demux/1 -> Mux/32
